simulink model "corr_test"  (Simulink 7.3)
settings: Solver=ode45  StartTime=0.0  StopTime=10000  RelTol=1e-3
libraries: xbsIndex_r4 x689, dali_library x32, dspsigops x2, xps_library x2, simulink x1, casper_library x1
(part 3 of 7)

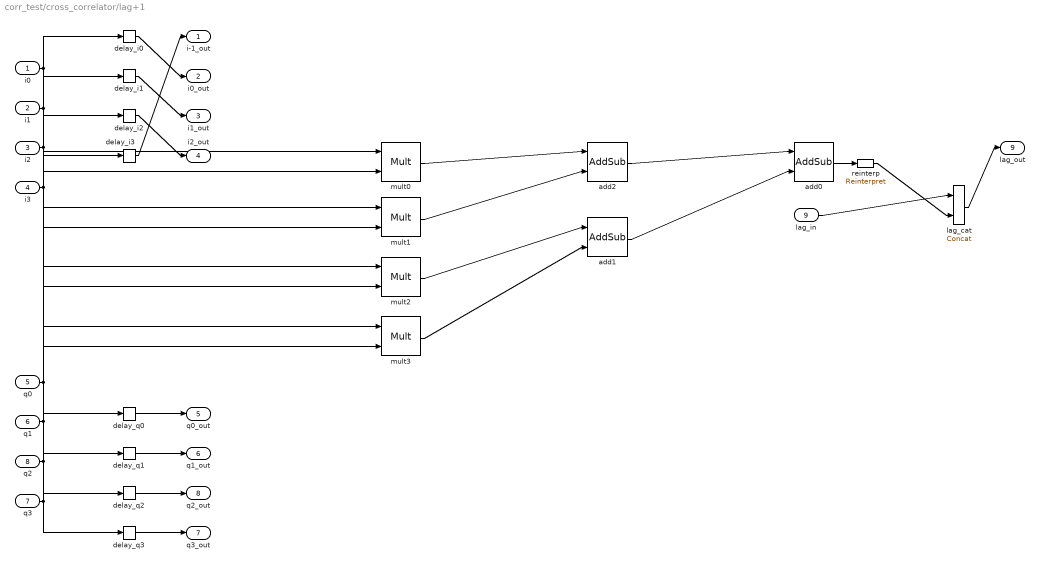
== system corr_test/cross_correlator/lag+1 ==
  i0 : Inport
  i1 : Inport  Port=2
  i2 : Inport  Port=3
  i3 : Inport  Port=4
  q0 : Inport  Port=5
  q1 : Inport  Port=6
  q3 : Inport  Port=7
  q2 : Inport  Port=8
  lag_in : Inport  Port=9
  add0 : xbsIndex_r4/AddSub  mode=Addition  use_carryin=off  use_carryout=off  en=off  latency=2  precision=Full  arith_type=Unsigned  n_bits=16  bin_pt=14  quantization=Truncate  overflow=Wrap  dbl_ovrd=off  use_behavioral_HDL=on  hw_selection=Fabric  pipelined=on  block_type=addsub
      settings: block_version=11.3
  add1 : xbsIndex_r4/AddSub  mode=Addition  use_carryin=off  use_carryout=off  en=off  latency=2  precision=Full  arith_type=Unsigned  n_bits=16  bin_pt=14  quantization=Truncate  overflow=Wrap  dbl_ovrd=off  use_behavioral_HDL=on  hw_selection=Fabric  pipelined=on  block_type=addsub
      settings: block_version=11.3
  add2 : xbsIndex_r4/AddSub  mode=Addition  use_carryin=off  use_carryout=off  en=off  latency=2  precision=Full  arith_type=Unsigned  n_bits=16  bin_pt=14  quantization=Truncate  overflow=Wrap  dbl_ovrd=off  use_behavioral_HDL=on  hw_selection=Fabric  pipelined=on  block_type=addsub
      settings: block_version=11.3
  delay_i0 : xbsIndex_r4/Delay  en=off  latency=0  dbl_ovrd=off  reg_retiming=off  block_type=delay
      settings: block_version=11.3
  delay_i1 : xbsIndex_r4/Delay  en=off  latency=0  dbl_ovrd=off  reg_retiming=off  block_type=delay
      settings: block_version=11.3
  delay_i2 : xbsIndex_r4/Delay  en=off  latency=0  dbl_ovrd=off  reg_retiming=off  block_type=delay
      settings: block_version=11.3
  delay_i3 : xbsIndex_r4/Delay  en=off  latency=1  dbl_ovrd=off  reg_retiming=off  block_type=delay
      settings: block_version=11.3
  delay_q{0..3} (4 alike) : xbsIndex_r4/Delay  en=off  latency=0  dbl_ovrd=off  reg_retiming=off  block_type=delay
      settings: block_version=11.3
  lag_cat : xbsIndex_r4/Concat  num_inputs=2  dbl_ovrd=off  block_type=concat
      settings: block_version=11.3
  mult{0..3} (4 alike) : xbsIndex_r4/Mult  precision=Full  arith_type="Signed  (2's comp)"  n_bits=16  bin_pt=14  quantization=Truncate  overflow=Wrap  en=off  latency=3  dbl_ovrd=off  use_behavioral_HDL=on  opt=Speed  use_embedded=off  optimum_pipeline=off  pipeline=on  use_rpm=on  placement_style=Triangular  block_type=mult
      settings: block_version=11.3
  reinterp : xbsIndex_r4/Reinterpret  force_arith_type=on  arith_type=Unsigned  force_bin_pt=on  bin_pt=0  block_type=reinterpret
      settings: infoedit="Changes signal type without altering the binary representation.   You can changed the signal between signed and unsigned, and relocate the binary point.<br><br>Hardware notes: In hardware this block costs nothing.<br><br>Example:  Suppose the input is 6 bits wide, signed, with 2 fractional bits, and the output is forced to unsigned with 0 fractional bits.  Then an input of -2.0 (1110.00 in binary 2's complement) becomes an output of 56 (111000 in binary)."  block_version=11.3
  i-1_out : Outport
  i0_out : Outport  Port=2
  i1_out : Outport  Port=3
  i2_out : Outport  Port=4
  q0_out : Outport  Port=5
  q1_out : Outport  Port=6
  q3_out : Outport  Port=7
  q2_out : Outport  Port=8
  lag_out : Outport  Port=9
  wires:
  i0/1 -> mult0/1, delay_i0/1
  q0/1 -> mult0/2, delay_q0/1
  i1/1 -> mult1/1, delay_i1/1
  q1/1 -> mult1/2, delay_q1/1
  i2/1 -> mult2/1, delay_i2/1
  q2/1 -> mult2/2, delay_q2/1
  i3/1 -> mult3/1, delay_i3/1
  q3/1 -> mult3/2, delay_q3/1
  mult0/1 -> add2/1
  mult1/1 -> add2/2
  mult2/1 -> add1/1
  mult3/1 -> add1/2
  add2/1 -> add0/1
  add1/1 -> add0/2
  delay_i0/1 -> i0_out/1
  delay_q0/1 -> q0_out/1
  delay_i1/1 -> i1_out/1
  delay_q1/1 -> q1_out/1
  delay_i2/1 -> i2_out/1
  delay_q2/1 -> q2_out/1
  delay_i3/1 -> i-1_out/1
  delay_q3/1 -> q3_out/1
  lag_in/1 -> lag_cat/1
  add0/1 -> reinterp/1
  reinterp/1 -> lag_cat/2
  lag_cat/1 -> lag_out/1

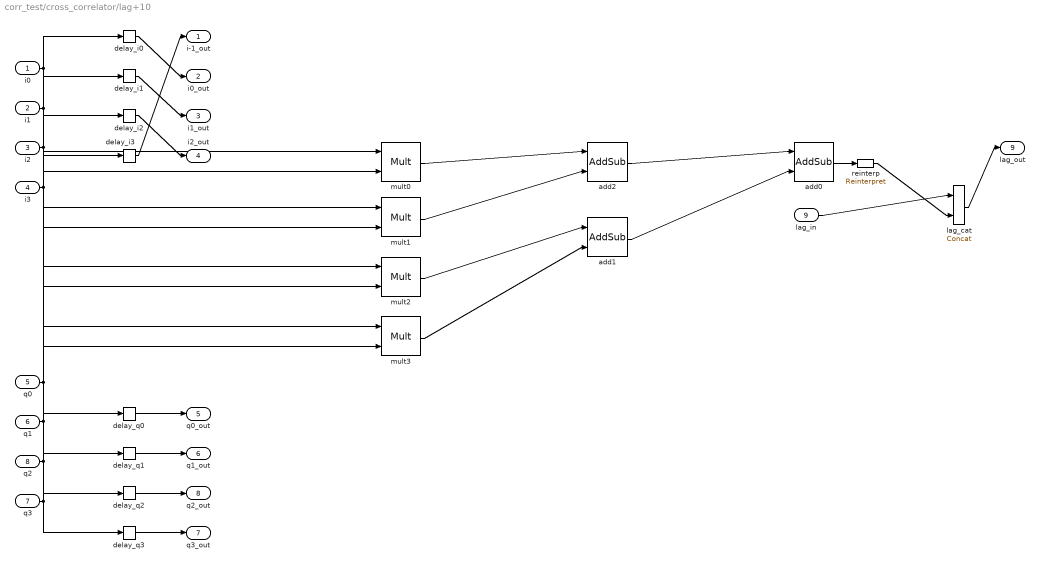
== system corr_test/cross_correlator/lag+10 ==
  i0 : Inport
  i1 : Inport  Port=2
  i2 : Inport  Port=3
  i3 : Inport  Port=4
  q0 : Inport  Port=5
  q1 : Inport  Port=6
  q3 : Inport  Port=7
  q2 : Inport  Port=8
  lag_in : Inport  Port=9
  add0 : xbsIndex_r4/AddSub  mode=Addition  use_carryin=off  use_carryout=off  en=off  latency=2  precision=Full  arith_type=Unsigned  n_bits=16  bin_pt=14  quantization=Truncate  overflow=Wrap  dbl_ovrd=off  use_behavioral_HDL=on  hw_selection=Fabric  pipelined=on  block_type=addsub
      settings: block_version=11.3
  add1 : xbsIndex_r4/AddSub  mode=Addition  use_carryin=off  use_carryout=off  en=off  latency=2  precision=Full  arith_type=Unsigned  n_bits=16  bin_pt=14  quantization=Truncate  overflow=Wrap  dbl_ovrd=off  use_behavioral_HDL=on  hw_selection=Fabric  pipelined=on  block_type=addsub
      settings: block_version=11.3
  add2 : xbsIndex_r4/AddSub  mode=Addition  use_carryin=off  use_carryout=off  en=off  latency=2  precision=Full  arith_type=Unsigned  n_bits=16  bin_pt=14  quantization=Truncate  overflow=Wrap  dbl_ovrd=off  use_behavioral_HDL=on  hw_selection=Fabric  pipelined=on  block_type=addsub
      settings: block_version=11.3
  delay_i0 : xbsIndex_r4/Delay  en=off  latency=0  dbl_ovrd=off  reg_retiming=off  block_type=delay
      settings: block_version=11.3
  delay_i1 : xbsIndex_r4/Delay  en=off  latency=0  dbl_ovrd=off  reg_retiming=off  block_type=delay
      settings: block_version=11.3
  delay_i2 : xbsIndex_r4/Delay  en=off  latency=0  dbl_ovrd=off  reg_retiming=off  block_type=delay
      settings: block_version=11.3
  delay_i3 : xbsIndex_r4/Delay  en=off  latency=1  dbl_ovrd=off  reg_retiming=off  block_type=delay
      settings: block_version=11.3
  delay_q{0..3} (4 alike) : xbsIndex_r4/Delay  en=off  latency=0  dbl_ovrd=off  reg_retiming=off  block_type=delay
      settings: block_version=11.3
  lag_cat : xbsIndex_r4/Concat  num_inputs=2  dbl_ovrd=off  block_type=concat
      settings: block_version=11.3
  mult{0..3} (4 alike) : xbsIndex_r4/Mult  precision=Full  arith_type="Signed  (2's comp)"  n_bits=16  bin_pt=14  quantization=Truncate  overflow=Wrap  en=off  latency=3  dbl_ovrd=off  use_behavioral_HDL=on  opt=Speed  use_embedded=off  optimum_pipeline=off  pipeline=on  use_rpm=on  placement_style=Triangular  block_type=mult
      settings: block_version=11.3
  reinterp : xbsIndex_r4/Reinterpret  force_arith_type=on  arith_type=Unsigned  force_bin_pt=on  bin_pt=0  block_type=reinterpret
      settings: infoedit="Changes signal type without altering the binary representation.   You can changed the signal between signed and unsigned, and relocate the binary point.<br><br>Hardware notes: In hardware this block costs nothing.<br><br>Example:  Suppose the input is 6 bits wide, signed, with 2 fractional bits, and the output is forced to unsigned with 0 fractional bits.  Then an input of -2.0 (1110.00 in binary 2's complement) becomes an output of 56 (111000 in binary)."  block_version=11.3
  i-1_out : Outport
  i0_out : Outport  Port=2
  i1_out : Outport  Port=3
  i2_out : Outport  Port=4
  q0_out : Outport  Port=5
  q1_out : Outport  Port=6
  q3_out : Outport  Port=7
  q2_out : Outport  Port=8
  lag_out : Outport  Port=9
  wires:
  i0/1 -> mult0/1, delay_i0/1
  q0/1 -> mult0/2, delay_q0/1
  i1/1 -> mult1/1, delay_i1/1
  q1/1 -> mult1/2, delay_q1/1
  i2/1 -> mult2/1, delay_i2/1
  q2/1 -> mult2/2, delay_q2/1
  i3/1 -> mult3/1, delay_i3/1
  q3/1 -> mult3/2, delay_q3/1
  mult0/1 -> add2/1
  mult1/1 -> add2/2
  mult2/1 -> add1/1
  mult3/1 -> add1/2
  add2/1 -> add0/1
  add1/1 -> add0/2
  delay_i0/1 -> i0_out/1
  delay_q0/1 -> q0_out/1
  delay_i1/1 -> i1_out/1
  delay_q1/1 -> q1_out/1
  delay_i2/1 -> i2_out/1
  delay_q2/1 -> q2_out/1
  delay_i3/1 -> i-1_out/1
  delay_q3/1 -> q3_out/1
  lag_in/1 -> lag_cat/1
  add0/1 -> reinterp/1
  reinterp/1 -> lag_cat/2
  lag_cat/1 -> lag_out/1

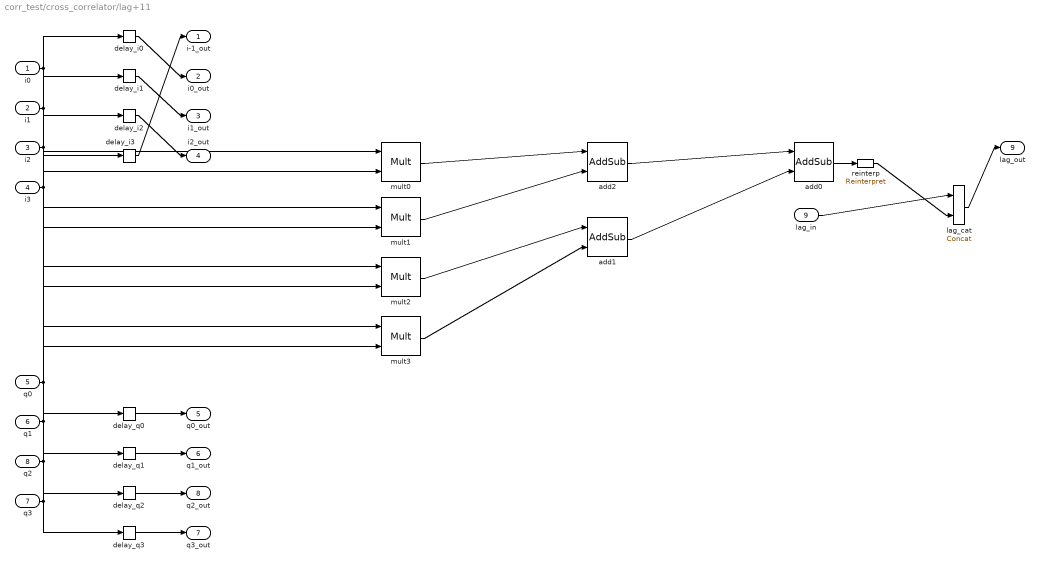
== system corr_test/cross_correlator/lag+11 ==
  i0 : Inport
  i1 : Inport  Port=2
  i2 : Inport  Port=3
  i3 : Inport  Port=4
  q0 : Inport  Port=5
  q1 : Inport  Port=6
  q3 : Inport  Port=7
  q2 : Inport  Port=8
  lag_in : Inport  Port=9
  add0 : xbsIndex_r4/AddSub  mode=Addition  use_carryin=off  use_carryout=off  en=off  latency=2  precision=Full  arith_type=Unsigned  n_bits=16  bin_pt=14  quantization=Truncate  overflow=Wrap  dbl_ovrd=off  use_behavioral_HDL=on  hw_selection=Fabric  pipelined=on  block_type=addsub
      settings: block_version=11.3
  add1 : xbsIndex_r4/AddSub  mode=Addition  use_carryin=off  use_carryout=off  en=off  latency=2  precision=Full  arith_type=Unsigned  n_bits=16  bin_pt=14  quantization=Truncate  overflow=Wrap  dbl_ovrd=off  use_behavioral_HDL=on  hw_selection=Fabric  pipelined=on  block_type=addsub
      settings: block_version=11.3
  add2 : xbsIndex_r4/AddSub  mode=Addition  use_carryin=off  use_carryout=off  en=off  latency=2  precision=Full  arith_type=Unsigned  n_bits=16  bin_pt=14  quantization=Truncate  overflow=Wrap  dbl_ovrd=off  use_behavioral_HDL=on  hw_selection=Fabric  pipelined=on  block_type=addsub
      settings: block_version=11.3
  delay_i0 : xbsIndex_r4/Delay  en=off  latency=0  dbl_ovrd=off  reg_retiming=off  block_type=delay
      settings: block_version=11.3
  delay_i1 : xbsIndex_r4/Delay  en=off  latency=0  dbl_ovrd=off  reg_retiming=off  block_type=delay
      settings: block_version=11.3
  delay_i2 : xbsIndex_r4/Delay  en=off  latency=0  dbl_ovrd=off  reg_retiming=off  block_type=delay
      settings: block_version=11.3
  delay_i3 : xbsIndex_r4/Delay  en=off  latency=1  dbl_ovrd=off  reg_retiming=off  block_type=delay
      settings: block_version=11.3
  delay_q{0..3} (4 alike) : xbsIndex_r4/Delay  en=off  latency=0  dbl_ovrd=off  reg_retiming=off  block_type=delay
      settings: block_version=11.3
  lag_cat : xbsIndex_r4/Concat  num_inputs=2  dbl_ovrd=off  block_type=concat
      settings: block_version=11.3
  mult{0..3} (4 alike) : xbsIndex_r4/Mult  precision=Full  arith_type="Signed  (2's comp)"  n_bits=16  bin_pt=14  quantization=Truncate  overflow=Wrap  en=off  latency=3  dbl_ovrd=off  use_behavioral_HDL=on  opt=Speed  use_embedded=off  optimum_pipeline=off  pipeline=on  use_rpm=on  placement_style=Triangular  block_type=mult
      settings: block_version=11.3
  reinterp : xbsIndex_r4/Reinterpret  force_arith_type=on  arith_type=Unsigned  force_bin_pt=on  bin_pt=0  block_type=reinterpret
      settings: infoedit="Changes signal type without altering the binary representation.   You can changed the signal between signed and unsigned, and relocate the binary point.<br><br>Hardware notes: In hardware this block costs nothing.<br><br>Example:  Suppose the input is 6 bits wide, signed, with 2 fractional bits, and the output is forced to unsigned with 0 fractional bits.  Then an input of -2.0 (1110.00 in binary 2's complement) becomes an output of 56 (111000 in binary)."  block_version=11.3
  i-1_out : Outport
  i0_out : Outport  Port=2
  i1_out : Outport  Port=3
  i2_out : Outport  Port=4
  q0_out : Outport  Port=5
  q1_out : Outport  Port=6
  q3_out : Outport  Port=7
  q2_out : Outport  Port=8
  lag_out : Outport  Port=9
  wires:
  i0/1 -> mult0/1, delay_i0/1
  q0/1 -> mult0/2, delay_q0/1
  i1/1 -> mult1/1, delay_i1/1
  q1/1 -> mult1/2, delay_q1/1
  i2/1 -> mult2/1, delay_i2/1
  q2/1 -> mult2/2, delay_q2/1
  i3/1 -> mult3/1, delay_i3/1
  q3/1 -> mult3/2, delay_q3/1
  mult0/1 -> add2/1
  mult1/1 -> add2/2
  mult2/1 -> add1/1
  mult3/1 -> add1/2
  add2/1 -> add0/1
  add1/1 -> add0/2
  delay_i0/1 -> i0_out/1
  delay_q0/1 -> q0_out/1
  delay_i1/1 -> i1_out/1
  delay_q1/1 -> q1_out/1
  delay_i2/1 -> i2_out/1
  delay_q2/1 -> q2_out/1
  delay_i3/1 -> i-1_out/1
  delay_q3/1 -> q3_out/1
  lag_in/1 -> lag_cat/1
  add0/1 -> reinterp/1
  reinterp/1 -> lag_cat/2
  lag_cat/1 -> lag_out/1

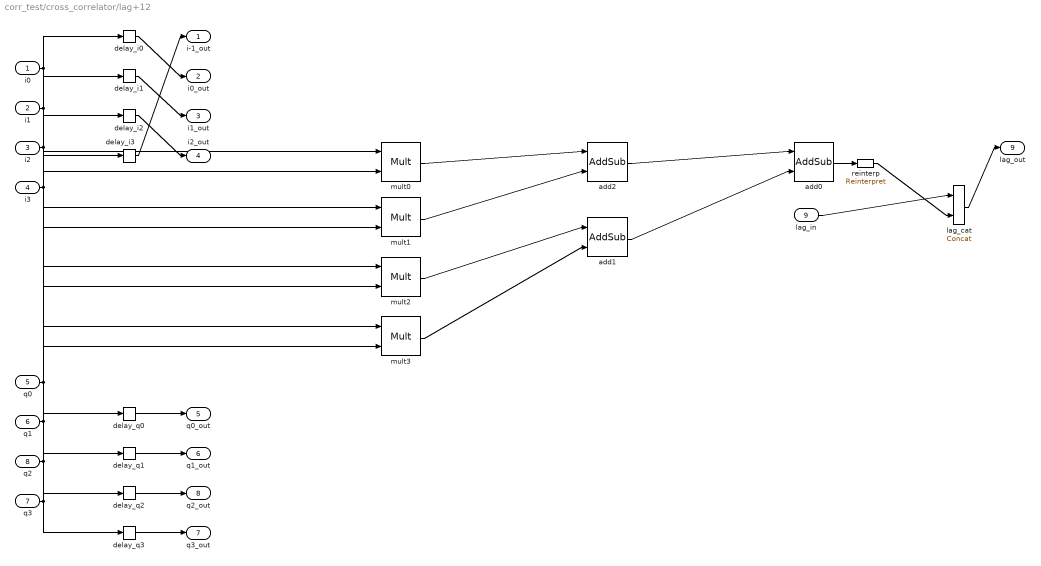
== system corr_test/cross_correlator/lag+12 ==
  i0 : Inport
  i1 : Inport  Port=2
  i2 : Inport  Port=3
  i3 : Inport  Port=4
  q0 : Inport  Port=5
  q1 : Inport  Port=6
  q3 : Inport  Port=7
  q2 : Inport  Port=8
  lag_in : Inport  Port=9
  add0 : xbsIndex_r4/AddSub  mode=Addition  use_carryin=off  use_carryout=off  en=off  latency=2  precision=Full  arith_type=Unsigned  n_bits=16  bin_pt=14  quantization=Truncate  overflow=Wrap  dbl_ovrd=off  use_behavioral_HDL=on  hw_selection=Fabric  pipelined=on  block_type=addsub
      settings: block_version=11.3
  add1 : xbsIndex_r4/AddSub  mode=Addition  use_carryin=off  use_carryout=off  en=off  latency=2  precision=Full  arith_type=Unsigned  n_bits=16  bin_pt=14  quantization=Truncate  overflow=Wrap  dbl_ovrd=off  use_behavioral_HDL=on  hw_selection=Fabric  pipelined=on  block_type=addsub
      settings: block_version=11.3
  add2 : xbsIndex_r4/AddSub  mode=Addition  use_carryin=off  use_carryout=off  en=off  latency=2  precision=Full  arith_type=Unsigned  n_bits=16  bin_pt=14  quantization=Truncate  overflow=Wrap  dbl_ovrd=off  use_behavioral_HDL=on  hw_selection=Fabric  pipelined=on  block_type=addsub
      settings: block_version=11.3
  delay_i0 : xbsIndex_r4/Delay  en=off  latency=0  dbl_ovrd=off  reg_retiming=off  block_type=delay
      settings: block_version=11.3
  delay_i1 : xbsIndex_r4/Delay  en=off  latency=0  dbl_ovrd=off  reg_retiming=off  block_type=delay
      settings: block_version=11.3
  delay_i2 : xbsIndex_r4/Delay  en=off  latency=0  dbl_ovrd=off  reg_retiming=off  block_type=delay
      settings: block_version=11.3
  delay_i3 : xbsIndex_r4/Delay  en=off  latency=1  dbl_ovrd=off  reg_retiming=off  block_type=delay
      settings: block_version=11.3
  delay_q{0..3} (4 alike) : xbsIndex_r4/Delay  en=off  latency=0  dbl_ovrd=off  reg_retiming=off  block_type=delay
      settings: block_version=11.3
  lag_cat : xbsIndex_r4/Concat  num_inputs=2  dbl_ovrd=off  block_type=concat
      settings: block_version=11.3
  mult{0..3} (4 alike) : xbsIndex_r4/Mult  precision=Full  arith_type="Signed  (2's comp)"  n_bits=16  bin_pt=14  quantization=Truncate  overflow=Wrap  en=off  latency=3  dbl_ovrd=off  use_behavioral_HDL=on  opt=Speed  use_embedded=off  optimum_pipeline=off  pipeline=on  use_rpm=on  placement_style=Triangular  block_type=mult
      settings: block_version=11.3
  reinterp : xbsIndex_r4/Reinterpret  force_arith_type=on  arith_type=Unsigned  force_bin_pt=on  bin_pt=0  block_type=reinterpret
      settings: infoedit="Changes signal type without altering the binary representation.   You can changed the signal between signed and unsigned, and relocate the binary point.<br><br>Hardware notes: In hardware this block costs nothing.<br><br>Example:  Suppose the input is 6 bits wide, signed, with 2 fractional bits, and the output is forced to unsigned with 0 fractional bits.  Then an input of -2.0 (1110.00 in binary 2's complement) becomes an output of 56 (111000 in binary)."  block_version=11.3
  i-1_out : Outport
  i0_out : Outport  Port=2
  i1_out : Outport  Port=3
  i2_out : Outport  Port=4
  q0_out : Outport  Port=5
  q1_out : Outport  Port=6
  q3_out : Outport  Port=7
  q2_out : Outport  Port=8
  lag_out : Outport  Port=9
  wires:
  i0/1 -> mult0/1, delay_i0/1
  q0/1 -> mult0/2, delay_q0/1
  i1/1 -> mult1/1, delay_i1/1
  q1/1 -> mult1/2, delay_q1/1
  i2/1 -> mult2/1, delay_i2/1
  q2/1 -> mult2/2, delay_q2/1
  i3/1 -> mult3/1, delay_i3/1
  q3/1 -> mult3/2, delay_q3/1
  mult0/1 -> add2/1
  mult1/1 -> add2/2
  mult2/1 -> add1/1
  mult3/1 -> add1/2
  add2/1 -> add0/1
  add1/1 -> add0/2
  delay_i0/1 -> i0_out/1
  delay_q0/1 -> q0_out/1
  delay_i1/1 -> i1_out/1
  delay_q1/1 -> q1_out/1
  delay_i2/1 -> i2_out/1
  delay_q2/1 -> q2_out/1
  delay_i3/1 -> i-1_out/1
  delay_q3/1 -> q3_out/1
  lag_in/1 -> lag_cat/1
  add0/1 -> reinterp/1
  reinterp/1 -> lag_cat/2
  lag_cat/1 -> lag_out/1

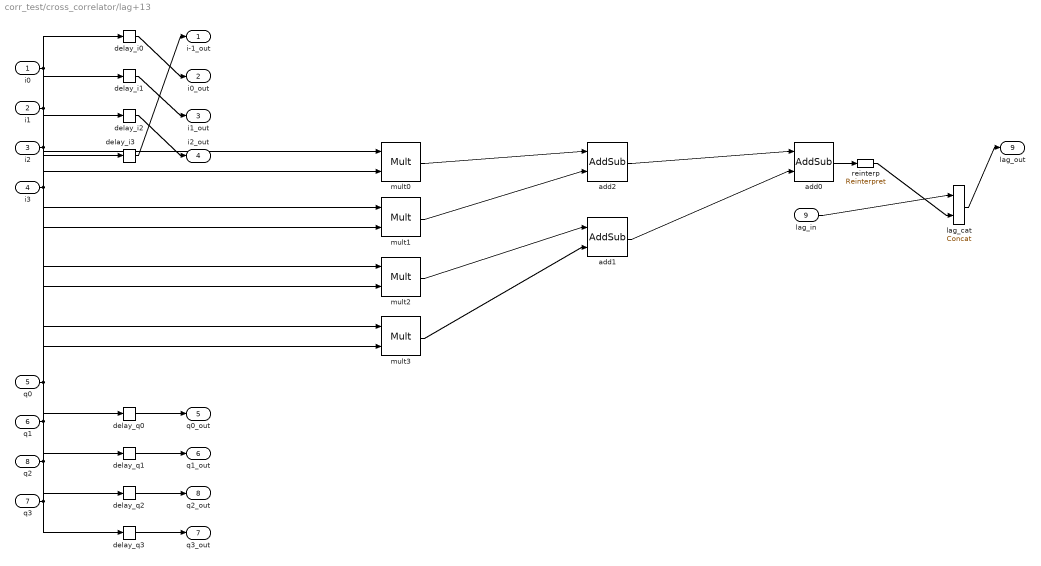
== system corr_test/cross_correlator/lag+13 ==
  i0 : Inport
  i1 : Inport  Port=2
  i2 : Inport  Port=3
  i3 : Inport  Port=4
  q0 : Inport  Port=5
  q1 : Inport  Port=6
  q3 : Inport  Port=7
  q2 : Inport  Port=8
  lag_in : Inport  Port=9
  add0 : xbsIndex_r4/AddSub  mode=Addition  use_carryin=off  use_carryout=off  en=off  latency=2  precision=Full  arith_type=Unsigned  n_bits=16  bin_pt=14  quantization=Truncate  overflow=Wrap  dbl_ovrd=off  use_behavioral_HDL=on  hw_selection=Fabric  pipelined=on  block_type=addsub
      settings: block_version=11.3
  add1 : xbsIndex_r4/AddSub  mode=Addition  use_carryin=off  use_carryout=off  en=off  latency=2  precision=Full  arith_type=Unsigned  n_bits=16  bin_pt=14  quantization=Truncate  overflow=Wrap  dbl_ovrd=off  use_behavioral_HDL=on  hw_selection=Fabric  pipelined=on  block_type=addsub
      settings: block_version=11.3
  add2 : xbsIndex_r4/AddSub  mode=Addition  use_carryin=off  use_carryout=off  en=off  latency=2  precision=Full  arith_type=Unsigned  n_bits=16  bin_pt=14  quantization=Truncate  overflow=Wrap  dbl_ovrd=off  use_behavioral_HDL=on  hw_selection=Fabric  pipelined=on  block_type=addsub
      settings: block_version=11.3
  delay_i0 : xbsIndex_r4/Delay  en=off  latency=0  dbl_ovrd=off  reg_retiming=off  block_type=delay
      settings: block_version=11.3
  delay_i1 : xbsIndex_r4/Delay  en=off  latency=0  dbl_ovrd=off  reg_retiming=off  block_type=delay
      settings: block_version=11.3
  delay_i2 : xbsIndex_r4/Delay  en=off  latency=0  dbl_ovrd=off  reg_retiming=off  block_type=delay
      settings: block_version=11.3
  delay_i3 : xbsIndex_r4/Delay  en=off  latency=1  dbl_ovrd=off  reg_retiming=off  block_type=delay
      settings: block_version=11.3
  delay_q{0..3} (4 alike) : xbsIndex_r4/Delay  en=off  latency=0  dbl_ovrd=off  reg_retiming=off  block_type=delay
      settings: block_version=11.3
  lag_cat : xbsIndex_r4/Concat  num_inputs=2  dbl_ovrd=off  block_type=concat
      settings: block_version=11.3
  mult{0..3} (4 alike) : xbsIndex_r4/Mult  precision=Full  arith_type="Signed  (2's comp)"  n_bits=16  bin_pt=14  quantization=Truncate  overflow=Wrap  en=off  latency=3  dbl_ovrd=off  use_behavioral_HDL=on  opt=Speed  use_embedded=off  optimum_pipeline=off  pipeline=on  use_rpm=on  placement_style=Triangular  block_type=mult
      settings: block_version=11.3
  reinterp : xbsIndex_r4/Reinterpret  force_arith_type=on  arith_type=Unsigned  force_bin_pt=on  bin_pt=0  block_type=reinterpret
      settings: infoedit="Changes signal type without altering the binary representation.   You can changed the signal between signed and unsigned, and relocate the binary point.<br><br>Hardware notes: In hardware this block costs nothing.<br><br>Example:  Suppose the input is 6 bits wide, signed, with 2 fractional bits, and the output is forced to unsigned with 0 fractional bits.  Then an input of -2.0 (1110.00 in binary 2's complement) becomes an output of 56 (111000 in binary)."  block_version=11.3
  i-1_out : Outport
  i0_out : Outport  Port=2
  i1_out : Outport  Port=3
  i2_out : Outport  Port=4
  q0_out : Outport  Port=5
  q1_out : Outport  Port=6
  q3_out : Outport  Port=7
  q2_out : Outport  Port=8
  lag_out : Outport  Port=9
  wires:
  i0/1 -> mult0/1, delay_i0/1
  q0/1 -> mult0/2, delay_q0/1
  i1/1 -> mult1/1, delay_i1/1
  q1/1 -> mult1/2, delay_q1/1
  i2/1 -> mult2/1, delay_i2/1
  q2/1 -> mult2/2, delay_q2/1
  i3/1 -> mult3/1, delay_i3/1
  q3/1 -> mult3/2, delay_q3/1
  mult0/1 -> add2/1
  mult1/1 -> add2/2
  mult2/1 -> add1/1
  mult3/1 -> add1/2
  add2/1 -> add0/1
  add1/1 -> add0/2
  delay_i0/1 -> i0_out/1
  delay_q0/1 -> q0_out/1
  delay_i1/1 -> i1_out/1
  delay_q1/1 -> q1_out/1
  delay_i2/1 -> i2_out/1
  delay_q2/1 -> q2_out/1
  delay_i3/1 -> i-1_out/1
  delay_q3/1 -> q3_out/1
  lag_in/1 -> lag_cat/1
  add0/1 -> reinterp/1
  reinterp/1 -> lag_cat/2
  lag_cat/1 -> lag_out/1

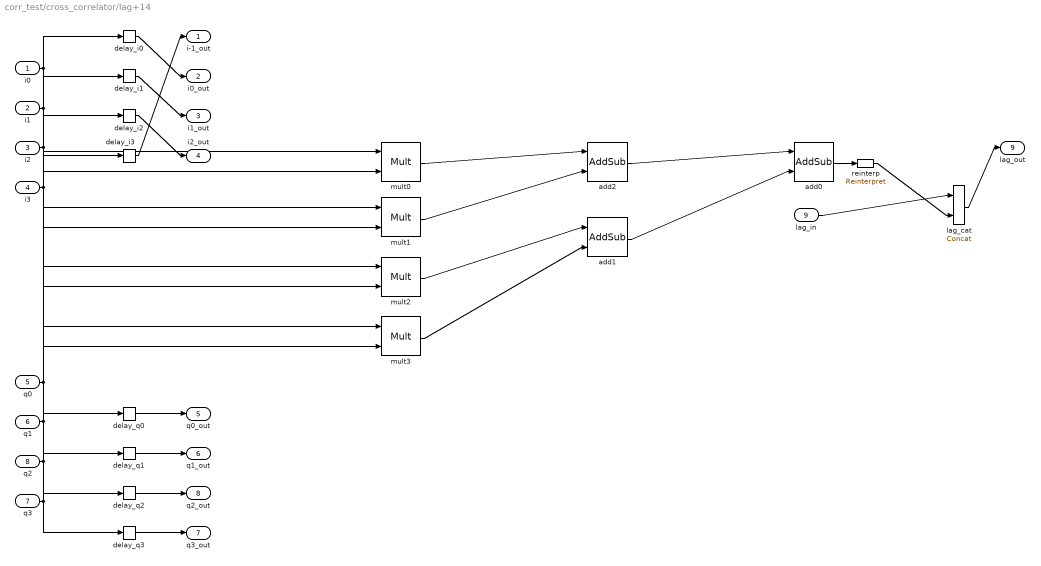
== system corr_test/cross_correlator/lag+14 ==
  i0 : Inport
  i1 : Inport  Port=2
  i2 : Inport  Port=3
  i3 : Inport  Port=4
  q0 : Inport  Port=5
  q1 : Inport  Port=6
  q3 : Inport  Port=7
  q2 : Inport  Port=8
  lag_in : Inport  Port=9
  add0 : xbsIndex_r4/AddSub  mode=Addition  use_carryin=off  use_carryout=off  en=off  latency=2  precision=Full  arith_type=Unsigned  n_bits=16  bin_pt=14  quantization=Truncate  overflow=Wrap  dbl_ovrd=off  use_behavioral_HDL=on  hw_selection=Fabric  pipelined=on  block_type=addsub
      settings: block_version=11.3
  add1 : xbsIndex_r4/AddSub  mode=Addition  use_carryin=off  use_carryout=off  en=off  latency=2  precision=Full  arith_type=Unsigned  n_bits=16  bin_pt=14  quantization=Truncate  overflow=Wrap  dbl_ovrd=off  use_behavioral_HDL=on  hw_selection=Fabric  pipelined=on  block_type=addsub
      settings: block_version=11.3
  add2 : xbsIndex_r4/AddSub  mode=Addition  use_carryin=off  use_carryout=off  en=off  latency=2  precision=Full  arith_type=Unsigned  n_bits=16  bin_pt=14  quantization=Truncate  overflow=Wrap  dbl_ovrd=off  use_behavioral_HDL=on  hw_selection=Fabric  pipelined=on  block_type=addsub
      settings: block_version=11.3
  delay_i0 : xbsIndex_r4/Delay  en=off  latency=0  dbl_ovrd=off  reg_retiming=off  block_type=delay
      settings: block_version=11.3
  delay_i1 : xbsIndex_r4/Delay  en=off  latency=0  dbl_ovrd=off  reg_retiming=off  block_type=delay
      settings: block_version=11.3
  delay_i2 : xbsIndex_r4/Delay  en=off  latency=0  dbl_ovrd=off  reg_retiming=off  block_type=delay
      settings: block_version=11.3
  delay_i3 : xbsIndex_r4/Delay  en=off  latency=1  dbl_ovrd=off  reg_retiming=off  block_type=delay
      settings: block_version=11.3
  delay_q{0..3} (4 alike) : xbsIndex_r4/Delay  en=off  latency=0  dbl_ovrd=off  reg_retiming=off  block_type=delay
      settings: block_version=11.3
  lag_cat : xbsIndex_r4/Concat  num_inputs=2  dbl_ovrd=off  block_type=concat
      settings: block_version=11.3
  mult{0..3} (4 alike) : xbsIndex_r4/Mult  precision=Full  arith_type="Signed  (2's comp)"  n_bits=16  bin_pt=14  quantization=Truncate  overflow=Wrap  en=off  latency=3  dbl_ovrd=off  use_behavioral_HDL=on  opt=Speed  use_embedded=off  optimum_pipeline=off  pipeline=on  use_rpm=on  placement_style=Triangular  block_type=mult
      settings: block_version=11.3
  reinterp : xbsIndex_r4/Reinterpret  force_arith_type=on  arith_type=Unsigned  force_bin_pt=on  bin_pt=0  block_type=reinterpret
      settings: infoedit="Changes signal type without altering the binary representation.   You can changed the signal between signed and unsigned, and relocate the binary point.<br><br>Hardware notes: In hardware this block costs nothing.<br><br>Example:  Suppose the input is 6 bits wide, signed, with 2 fractional bits, and the output is forced to unsigned with 0 fractional bits.  Then an input of -2.0 (1110.00 in binary 2's complement) becomes an output of 56 (111000 in binary)."  block_version=11.3
  i-1_out : Outport
  i0_out : Outport  Port=2
  i1_out : Outport  Port=3
  i2_out : Outport  Port=4
  q0_out : Outport  Port=5
  q1_out : Outport  Port=6
  q3_out : Outport  Port=7
  q2_out : Outport  Port=8
  lag_out : Outport  Port=9
  wires:
  i0/1 -> mult0/1, delay_i0/1
  q0/1 -> mult0/2, delay_q0/1
  i1/1 -> mult1/1, delay_i1/1
  q1/1 -> mult1/2, delay_q1/1
  i2/1 -> mult2/1, delay_i2/1
  q2/1 -> mult2/2, delay_q2/1
  i3/1 -> mult3/1, delay_i3/1
  q3/1 -> mult3/2, delay_q3/1
  mult0/1 -> add2/1
  mult1/1 -> add2/2
  mult2/1 -> add1/1
  mult3/1 -> add1/2
  add2/1 -> add0/1
  add1/1 -> add0/2
  delay_i0/1 -> i0_out/1
  delay_q0/1 -> q0_out/1
  delay_i1/1 -> i1_out/1
  delay_q1/1 -> q1_out/1
  delay_i2/1 -> i2_out/1
  delay_q2/1 -> q2_out/1
  delay_i3/1 -> i-1_out/1
  delay_q3/1 -> q3_out/1
  lag_in/1 -> lag_cat/1
  add0/1 -> reinterp/1
  reinterp/1 -> lag_cat/2
  lag_cat/1 -> lag_out/1

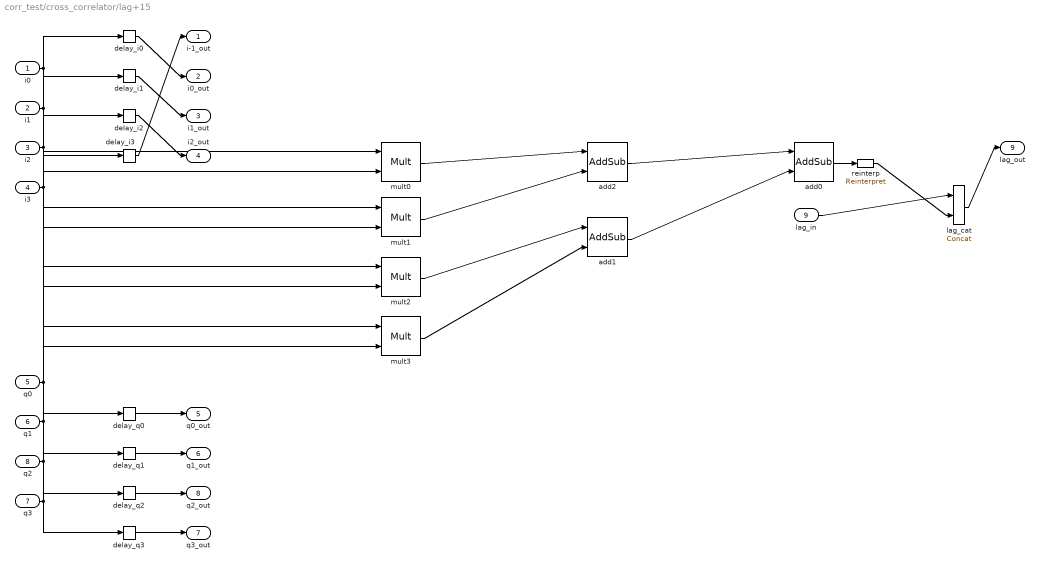
== system corr_test/cross_correlator/lag+15 ==
  i0 : Inport
  i1 : Inport  Port=2
  i2 : Inport  Port=3
  i3 : Inport  Port=4
  q0 : Inport  Port=5
  q1 : Inport  Port=6
  q3 : Inport  Port=7
  q2 : Inport  Port=8
  lag_in : Inport  Port=9
  add0 : xbsIndex_r4/AddSub  mode=Addition  use_carryin=off  use_carryout=off  en=off  latency=2  precision=Full  arith_type=Unsigned  n_bits=16  bin_pt=14  quantization=Truncate  overflow=Wrap  dbl_ovrd=off  use_behavioral_HDL=on  hw_selection=Fabric  pipelined=on  block_type=addsub
      settings: block_version=11.3
  add1 : xbsIndex_r4/AddSub  mode=Addition  use_carryin=off  use_carryout=off  en=off  latency=2  precision=Full  arith_type=Unsigned  n_bits=16  bin_pt=14  quantization=Truncate  overflow=Wrap  dbl_ovrd=off  use_behavioral_HDL=on  hw_selection=Fabric  pipelined=on  block_type=addsub
      settings: block_version=11.3
  add2 : xbsIndex_r4/AddSub  mode=Addition  use_carryin=off  use_carryout=off  en=off  latency=2  precision=Full  arith_type=Unsigned  n_bits=16  bin_pt=14  quantization=Truncate  overflow=Wrap  dbl_ovrd=off  use_behavioral_HDL=on  hw_selection=Fabric  pipelined=on  block_type=addsub
      settings: block_version=11.3
  delay_i0 : xbsIndex_r4/Delay  en=off  latency=0  dbl_ovrd=off  reg_retiming=off  block_type=delay
      settings: block_version=11.3
  delay_i1 : xbsIndex_r4/Delay  en=off  latency=0  dbl_ovrd=off  reg_retiming=off  block_type=delay
      settings: block_version=11.3
  delay_i2 : xbsIndex_r4/Delay  en=off  latency=0  dbl_ovrd=off  reg_retiming=off  block_type=delay
      settings: block_version=11.3
  delay_i3 : xbsIndex_r4/Delay  en=off  latency=1  dbl_ovrd=off  reg_retiming=off  block_type=delay
      settings: block_version=11.3
  delay_q{0..3} (4 alike) : xbsIndex_r4/Delay  en=off  latency=0  dbl_ovrd=off  reg_retiming=off  block_type=delay
      settings: block_version=11.3
  lag_cat : xbsIndex_r4/Concat  num_inputs=2  dbl_ovrd=off  block_type=concat
      settings: block_version=11.3
  mult{0..3} (4 alike) : xbsIndex_r4/Mult  precision=Full  arith_type="Signed  (2's comp)"  n_bits=16  bin_pt=14  quantization=Truncate  overflow=Wrap  en=off  latency=3  dbl_ovrd=off  use_behavioral_HDL=on  opt=Speed  use_embedded=off  optimum_pipeline=off  pipeline=on  use_rpm=on  placement_style=Triangular  block_type=mult
      settings: block_version=11.3
  reinterp : xbsIndex_r4/Reinterpret  force_arith_type=on  arith_type=Unsigned  force_bin_pt=on  bin_pt=0  block_type=reinterpret
      settings: infoedit="Changes signal type without altering the binary representation.   You can changed the signal between signed and unsigned, and relocate the binary point.<br><br>Hardware notes: In hardware this block costs nothing.<br><br>Example:  Suppose the input is 6 bits wide, signed, with 2 fractional bits, and the output is forced to unsigned with 0 fractional bits.  Then an input of -2.0 (1110.00 in binary 2's complement) becomes an output of 56 (111000 in binary)."  block_version=11.3
  i-1_out : Outport
  i0_out : Outport  Port=2
  i1_out : Outport  Port=3
  i2_out : Outport  Port=4
  q0_out : Outport  Port=5
  q1_out : Outport  Port=6
  q3_out : Outport  Port=7
  q2_out : Outport  Port=8
  lag_out : Outport  Port=9
  wires:
  i0/1 -> mult0/1, delay_i0/1
  q0/1 -> mult0/2, delay_q0/1
  i1/1 -> mult1/1, delay_i1/1
  q1/1 -> mult1/2, delay_q1/1
  i2/1 -> mult2/1, delay_i2/1
  q2/1 -> mult2/2, delay_q2/1
  i3/1 -> mult3/1, delay_i3/1
  q3/1 -> mult3/2, delay_q3/1
  mult0/1 -> add2/1
  mult1/1 -> add2/2
  mult2/1 -> add1/1
  mult3/1 -> add1/2
  add2/1 -> add0/1
  add1/1 -> add0/2
  delay_i0/1 -> i0_out/1
  delay_q0/1 -> q0_out/1
  delay_i1/1 -> i1_out/1
  delay_q1/1 -> q1_out/1
  delay_i2/1 -> i2_out/1
  delay_q2/1 -> q2_out/1
  delay_i3/1 -> i-1_out/1
  delay_q3/1 -> q3_out/1
  lag_in/1 -> lag_cat/1
  add0/1 -> reinterp/1
  reinterp/1 -> lag_cat/2
  lag_cat/1 -> lag_out/1

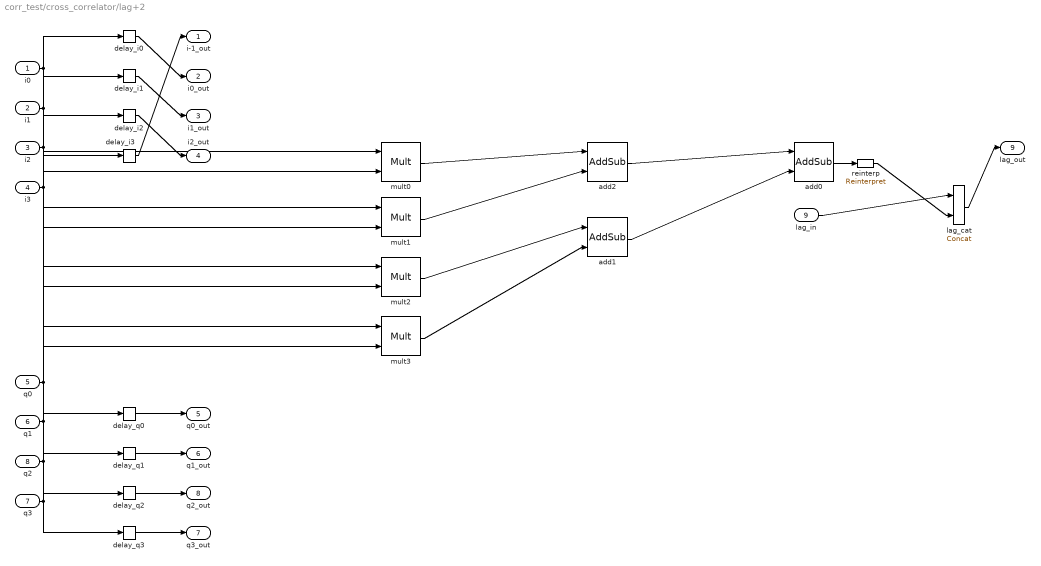
== system corr_test/cross_correlator/lag+2 ==
  i0 : Inport
  i1 : Inport  Port=2
  i2 : Inport  Port=3
  i3 : Inport  Port=4
  q0 : Inport  Port=5
  q1 : Inport  Port=6
  q3 : Inport  Port=7
  q2 : Inport  Port=8
  lag_in : Inport  Port=9
  add0 : xbsIndex_r4/AddSub  mode=Addition  use_carryin=off  use_carryout=off  en=off  latency=2  precision=Full  arith_type=Unsigned  n_bits=16  bin_pt=14  quantization=Truncate  overflow=Wrap  dbl_ovrd=off  use_behavioral_HDL=on  hw_selection=Fabric  pipelined=on  block_type=addsub
      settings: block_version=11.3
  add1 : xbsIndex_r4/AddSub  mode=Addition  use_carryin=off  use_carryout=off  en=off  latency=2  precision=Full  arith_type=Unsigned  n_bits=16  bin_pt=14  quantization=Truncate  overflow=Wrap  dbl_ovrd=off  use_behavioral_HDL=on  hw_selection=Fabric  pipelined=on  block_type=addsub
      settings: block_version=11.3
  add2 : xbsIndex_r4/AddSub  mode=Addition  use_carryin=off  use_carryout=off  en=off  latency=2  precision=Full  arith_type=Unsigned  n_bits=16  bin_pt=14  quantization=Truncate  overflow=Wrap  dbl_ovrd=off  use_behavioral_HDL=on  hw_selection=Fabric  pipelined=on  block_type=addsub
      settings: block_version=11.3
  delay_i0 : xbsIndex_r4/Delay  en=off  latency=0  dbl_ovrd=off  reg_retiming=off  block_type=delay
      settings: block_version=11.3
  delay_i1 : xbsIndex_r4/Delay  en=off  latency=0  dbl_ovrd=off  reg_retiming=off  block_type=delay
      settings: block_version=11.3
  delay_i2 : xbsIndex_r4/Delay  en=off  latency=0  dbl_ovrd=off  reg_retiming=off  block_type=delay
      settings: block_version=11.3
  delay_i3 : xbsIndex_r4/Delay  en=off  latency=1  dbl_ovrd=off  reg_retiming=off  block_type=delay
      settings: block_version=11.3
  delay_q{0..3} (4 alike) : xbsIndex_r4/Delay  en=off  latency=0  dbl_ovrd=off  reg_retiming=off  block_type=delay
      settings: block_version=11.3
  lag_cat : xbsIndex_r4/Concat  num_inputs=2  dbl_ovrd=off  block_type=concat
      settings: block_version=11.3
  mult{0..3} (4 alike) : xbsIndex_r4/Mult  precision=Full  arith_type="Signed  (2's comp)"  n_bits=16  bin_pt=14  quantization=Truncate  overflow=Wrap  en=off  latency=3  dbl_ovrd=off  use_behavioral_HDL=on  opt=Speed  use_embedded=off  optimum_pipeline=off  pipeline=on  use_rpm=on  placement_style=Triangular  block_type=mult
      settings: block_version=11.3
  reinterp : xbsIndex_r4/Reinterpret  force_arith_type=on  arith_type=Unsigned  force_bin_pt=on  bin_pt=0  block_type=reinterpret
      settings: infoedit="Changes signal type without altering the binary representation.   You can changed the signal between signed and unsigned, and relocate the binary point.<br><br>Hardware notes: In hardware this block costs nothing.<br><br>Example:  Suppose the input is 6 bits wide, signed, with 2 fractional bits, and the output is forced to unsigned with 0 fractional bits.  Then an input of -2.0 (1110.00 in binary 2's complement) becomes an output of 56 (111000 in binary)."  block_version=11.3
  i-1_out : Outport
  i0_out : Outport  Port=2
  i1_out : Outport  Port=3
  i2_out : Outport  Port=4
  q0_out : Outport  Port=5
  q1_out : Outport  Port=6
  q3_out : Outport  Port=7
  q2_out : Outport  Port=8
  lag_out : Outport  Port=9
  wires:
  i0/1 -> mult0/1, delay_i0/1
  q0/1 -> mult0/2, delay_q0/1
  i1/1 -> mult1/1, delay_i1/1
  q1/1 -> mult1/2, delay_q1/1
  i2/1 -> mult2/1, delay_i2/1
  q2/1 -> mult2/2, delay_q2/1
  i3/1 -> mult3/1, delay_i3/1
  q3/1 -> mult3/2, delay_q3/1
  mult0/1 -> add2/1
  mult1/1 -> add2/2
  mult2/1 -> add1/1
  mult3/1 -> add1/2
  add2/1 -> add0/1
  add1/1 -> add0/2
  delay_i0/1 -> i0_out/1
  delay_q0/1 -> q0_out/1
  delay_i1/1 -> i1_out/1
  delay_q1/1 -> q1_out/1
  delay_i2/1 -> i2_out/1
  delay_q2/1 -> q2_out/1
  delay_i3/1 -> i-1_out/1
  delay_q3/1 -> q3_out/1
  lag_in/1 -> lag_cat/1
  add0/1 -> reinterp/1
  reinterp/1 -> lag_cat/2
  lag_cat/1 -> lag_out/1

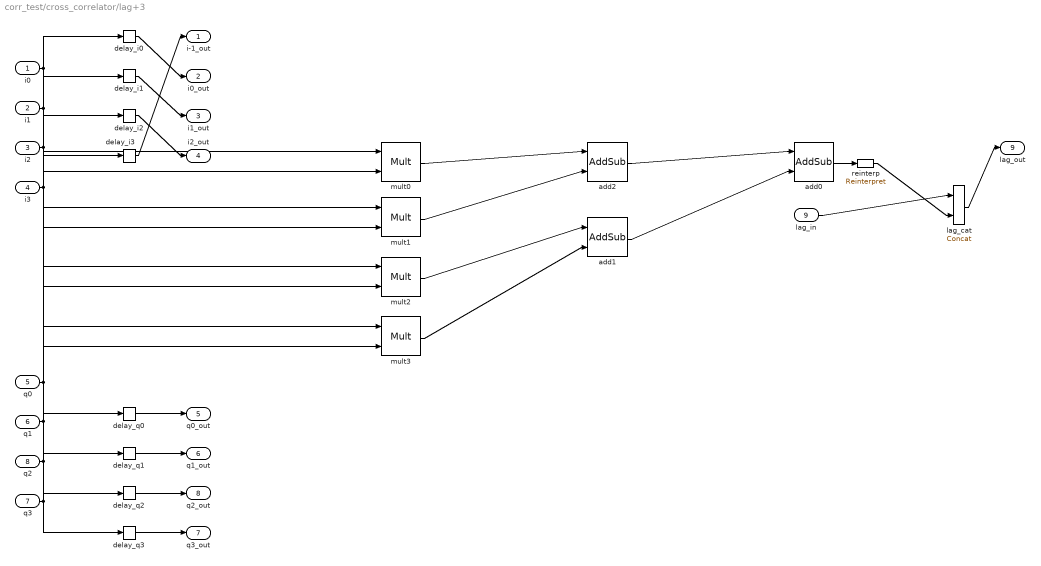
== system corr_test/cross_correlator/lag+3 ==
  i0 : Inport
  i1 : Inport  Port=2
  i2 : Inport  Port=3
  i3 : Inport  Port=4
  q0 : Inport  Port=5
  q1 : Inport  Port=6
  q3 : Inport  Port=7
  q2 : Inport  Port=8
  lag_in : Inport  Port=9
  add0 : xbsIndex_r4/AddSub  mode=Addition  use_carryin=off  use_carryout=off  en=off  latency=2  precision=Full  arith_type=Unsigned  n_bits=16  bin_pt=14  quantization=Truncate  overflow=Wrap  dbl_ovrd=off  use_behavioral_HDL=on  hw_selection=Fabric  pipelined=on  block_type=addsub
      settings: block_version=11.3
  add1 : xbsIndex_r4/AddSub  mode=Addition  use_carryin=off  use_carryout=off  en=off  latency=2  precision=Full  arith_type=Unsigned  n_bits=16  bin_pt=14  quantization=Truncate  overflow=Wrap  dbl_ovrd=off  use_behavioral_HDL=on  hw_selection=Fabric  pipelined=on  block_type=addsub
      settings: block_version=11.3
  add2 : xbsIndex_r4/AddSub  mode=Addition  use_carryin=off  use_carryout=off  en=off  latency=2  precision=Full  arith_type=Unsigned  n_bits=16  bin_pt=14  quantization=Truncate  overflow=Wrap  dbl_ovrd=off  use_behavioral_HDL=on  hw_selection=Fabric  pipelined=on  block_type=addsub
      settings: block_version=11.3
  delay_i0 : xbsIndex_r4/Delay  en=off  latency=0  dbl_ovrd=off  reg_retiming=off  block_type=delay
      settings: block_version=11.3
  delay_i1 : xbsIndex_r4/Delay  en=off  latency=0  dbl_ovrd=off  reg_retiming=off  block_type=delay
      settings: block_version=11.3
  delay_i2 : xbsIndex_r4/Delay  en=off  latency=0  dbl_ovrd=off  reg_retiming=off  block_type=delay
      settings: block_version=11.3
  delay_i3 : xbsIndex_r4/Delay  en=off  latency=1  dbl_ovrd=off  reg_retiming=off  block_type=delay
      settings: block_version=11.3
  delay_q{0..3} (4 alike) : xbsIndex_r4/Delay  en=off  latency=0  dbl_ovrd=off  reg_retiming=off  block_type=delay
      settings: block_version=11.3
  lag_cat : xbsIndex_r4/Concat  num_inputs=2  dbl_ovrd=off  block_type=concat
      settings: block_version=11.3
  mult{0..3} (4 alike) : xbsIndex_r4/Mult  precision=Full  arith_type="Signed  (2's comp)"  n_bits=16  bin_pt=14  quantization=Truncate  overflow=Wrap  en=off  latency=3  dbl_ovrd=off  use_behavioral_HDL=on  opt=Speed  use_embedded=off  optimum_pipeline=off  pipeline=on  use_rpm=on  placement_style=Triangular  block_type=mult
      settings: block_version=11.3
  reinterp : xbsIndex_r4/Reinterpret  force_arith_type=on  arith_type=Unsigned  force_bin_pt=on  bin_pt=0  block_type=reinterpret
      settings: infoedit="Changes signal type without altering the binary representation.   You can changed the signal between signed and unsigned, and relocate the binary point.<br><br>Hardware notes: In hardware this block costs nothing.<br><br>Example:  Suppose the input is 6 bits wide, signed, with 2 fractional bits, and the output is forced to unsigned with 0 fractional bits.  Then an input of -2.0 (1110.00 in binary 2's complement) becomes an output of 56 (111000 in binary)."  block_version=11.3
  i-1_out : Outport
  i0_out : Outport  Port=2
  i1_out : Outport  Port=3
  i2_out : Outport  Port=4
  q0_out : Outport  Port=5
  q1_out : Outport  Port=6
  q3_out : Outport  Port=7
  q2_out : Outport  Port=8
  lag_out : Outport  Port=9
  wires:
  i0/1 -> mult0/1, delay_i0/1
  q0/1 -> mult0/2, delay_q0/1
  i1/1 -> mult1/1, delay_i1/1
  q1/1 -> mult1/2, delay_q1/1
  i2/1 -> mult2/1, delay_i2/1
  q2/1 -> mult2/2, delay_q2/1
  i3/1 -> mult3/1, delay_i3/1
  q3/1 -> mult3/2, delay_q3/1
  mult0/1 -> add2/1
  mult1/1 -> add2/2
  mult2/1 -> add1/1
  mult3/1 -> add1/2
  add2/1 -> add0/1
  add1/1 -> add0/2
  delay_i0/1 -> i0_out/1
  delay_q0/1 -> q0_out/1
  delay_i1/1 -> i1_out/1
  delay_q1/1 -> q1_out/1
  delay_i2/1 -> i2_out/1
  delay_q2/1 -> q2_out/1
  delay_i3/1 -> i-1_out/1
  delay_q3/1 -> q3_out/1
  lag_in/1 -> lag_cat/1
  add0/1 -> reinterp/1
  reinterp/1 -> lag_cat/2
  lag_cat/1 -> lag_out/1

== system corr_test/cross_correlator/lag+4 ==
  i0 : Inport
  i1 : Inport  Port=2
  i2 : Inport  Port=3
  i3 : Inport  Port=4
  q0 : Inport  Port=5
  q1 : Inport  Port=6
  q3 : Inport  Port=7
  q2 : Inport  Port=8
  lag_in : Inport  Port=9
  add0 : xbsIndex_r4/AddSub  mode=Addition  use_carryin=off  use_carryout=off  en=off  latency=2  precision=Full  arith_type=Unsigned  n_bits=16  bin_pt=14  quantization=Truncate  overflow=Wrap  dbl_ovrd=off  use_behavioral_HDL=on  hw_selection=Fabric  pipelined=on  block_type=addsub
      settings: block_version=11.3
  add1 : xbsIndex_r4/AddSub  mode=Addition  use_carryin=off  use_carryout=off  en=off  latency=2  precision=Full  arith_type=Unsigned  n_bits=16  bin_pt=14  quantization=Truncate  overflow=Wrap  dbl_ovrd=off  use_behavioral_HDL=on  hw_selection=Fabric  pipelined=on  block_type=addsub
      settings: block_version=11.3
  add2 : xbsIndex_r4/AddSub  mode=Addition  use_carryin=off  use_carryout=off  en=off  latency=2  precision=Full  arith_type=Unsigned  n_bits=16  bin_pt=14  quantization=Truncate  overflow=Wrap  dbl_ovrd=off  use_behavioral_HDL=on  hw_selection=Fabric  pipelined=on  block_type=addsub
      settings: block_version=11.3
  delay_i0 : xbsIndex_r4/Delay  en=off  latency=0  dbl_ovrd=off  reg_retiming=off  block_type=delay
      settings: block_version=11.3
  delay_i1 : xbsIndex_r4/Delay  en=off  latency=0  dbl_ovrd=off  reg_retiming=off  block_type=delay
      settings: block_version=11.3
  delay_i2 : xbsIndex_r4/Delay  en=off  latency=0  dbl_ovrd=off  reg_retiming=off  block_type=delay
      settings: block_version=11.3
  delay_i3 : xbsIndex_r4/Delay  en=off  latency=1  dbl_ovrd=off  reg_retiming=off  block_type=delay
      settings: block_version=11.3
  delay_q{0..3} (4 alike) : xbsIndex_r4/Delay  en=off  latency=0  dbl_ovrd=off  reg_retiming=off  block_type=delay
      settings: block_version=11.3
  lag_cat : xbsIndex_r4/Concat  num_inputs=2  dbl_ovrd=off  block_type=concat
      settings: block_version=11.3
  mult{0..3} (4 alike) : xbsIndex_r4/Mult  precision=Full  arith_type="Signed  (2's comp)"  n_bits=16  bin_pt=14  quantization=Truncate  overflow=Wrap  en=off  latency=3  dbl_ovrd=off  use_behavioral_HDL=on  opt=Speed  use_embedded=off  optimum_pipeline=off  pipeline=on  use_rpm=on  placement_style=Triangular  block_type=mult
      settings: block_version=11.3
  reinterp : xbsIndex_r4/Reinterpret  force_arith_type=on  arith_type=Unsigned  force_bin_pt=on  bin_pt=0  block_type=reinterpret
      settings: infoedit="Changes signal type without altering the binary representation.   You can changed the signal between signed and unsigned, and relocate the binary point.<br><br>Hardware notes: In hardware this block costs nothing.<br><br>Example:  Suppose the input is 6 bits wide, signed, with 2 fractional bits, and the output is forced to unsigned with 0 fractional bits.  Then an input of -2.0 (1110.00 in binary 2's complement) becomes an output of 56 (111000 in binary)."  block_version=11.3
  i-1_out : Outport
  i0_out : Outport  Port=2
  i1_out : Outport  Port=3
  i2_out : Outport  Port=4
  q0_out : Outport  Port=5
  q1_out : Outport  Port=6
  q3_out : Outport  Port=7
  q2_out : Outport  Port=8
  lag_out : Outport  Port=9
  wires:
  i0/1 -> mult0/1, delay_i0/1
  q0/1 -> mult0/2, delay_q0/1
  i1/1 -> mult1/1, delay_i1/1
  q1/1 -> mult1/2, delay_q1/1
  i2/1 -> mult2/1, delay_i2/1
  q2/1 -> mult2/2, delay_q2/1
  i3/1 -> mult3/1, delay_i3/1
  q3/1 -> mult3/2, delay_q3/1
  mult0/1 -> add2/1
  mult1/1 -> add2/2
  mult2/1 -> add1/1
  mult3/1 -> add1/2
  add2/1 -> add0/1
  add1/1 -> add0/2
  delay_i0/1 -> i0_out/1
  delay_q0/1 -> q0_out/1
  delay_i1/1 -> i1_out/1
  delay_q1/1 -> q1_out/1
  delay_i2/1 -> i2_out/1
  delay_q2/1 -> q2_out/1
  delay_i3/1 -> i-1_out/1
  delay_q3/1 -> q3_out/1
  lag_in/1 -> lag_cat/1
  add0/1 -> reinterp/1
  reinterp/1 -> lag_cat/2
  lag_cat/1 -> lag_out/1

== system corr_test/cross_correlator/lag+5 ==
  i0 : Inport
  i1 : Inport  Port=2
  i2 : Inport  Port=3
  i3 : Inport  Port=4
  q0 : Inport  Port=5
  q1 : Inport  Port=6
  q3 : Inport  Port=7
  q2 : Inport  Port=8
  lag_in : Inport  Port=9
  add0 : xbsIndex_r4/AddSub  mode=Addition  use_carryin=off  use_carryout=off  en=off  latency=2  precision=Full  arith_type=Unsigned  n_bits=16  bin_pt=14  quantization=Truncate  overflow=Wrap  dbl_ovrd=off  use_behavioral_HDL=on  hw_selection=Fabric  pipelined=on  block_type=addsub
      settings: block_version=11.3
  add1 : xbsIndex_r4/AddSub  mode=Addition  use_carryin=off  use_carryout=off  en=off  latency=2  precision=Full  arith_type=Unsigned  n_bits=16  bin_pt=14  quantization=Truncate  overflow=Wrap  dbl_ovrd=off  use_behavioral_HDL=on  hw_selection=Fabric  pipelined=on  block_type=addsub
      settings: block_version=11.3
  add2 : xbsIndex_r4/AddSub  mode=Addition  use_carryin=off  use_carryout=off  en=off  latency=2  precision=Full  arith_type=Unsigned  n_bits=16  bin_pt=14  quantization=Truncate  overflow=Wrap  dbl_ovrd=off  use_behavioral_HDL=on  hw_selection=Fabric  pipelined=on  block_type=addsub
      settings: block_version=11.3
  delay_i0 : xbsIndex_r4/Delay  en=off  latency=0  dbl_ovrd=off  reg_retiming=off  block_type=delay
      settings: block_version=11.3
  delay_i1 : xbsIndex_r4/Delay  en=off  latency=0  dbl_ovrd=off  reg_retiming=off  block_type=delay
      settings: block_version=11.3
  delay_i2 : xbsIndex_r4/Delay  en=off  latency=0  dbl_ovrd=off  reg_retiming=off  block_type=delay
      settings: block_version=11.3
  delay_i3 : xbsIndex_r4/Delay  en=off  latency=1  dbl_ovrd=off  reg_retiming=off  block_type=delay
      settings: block_version=11.3
  delay_q{0..3} (4 alike) : xbsIndex_r4/Delay  en=off  latency=0  dbl_ovrd=off  reg_retiming=off  block_type=delay
      settings: block_version=11.3
  lag_cat : xbsIndex_r4/Concat  num_inputs=2  dbl_ovrd=off  block_type=concat
      settings: block_version=11.3
  mult{0..3} (4 alike) : xbsIndex_r4/Mult  precision=Full  arith_type="Signed  (2's comp)"  n_bits=16  bin_pt=14  quantization=Truncate  overflow=Wrap  en=off  latency=3  dbl_ovrd=off  use_behavioral_HDL=on  opt=Speed  use_embedded=off  optimum_pipeline=off  pipeline=on  use_rpm=on  placement_style=Triangular  block_type=mult
      settings: block_version=11.3
  reinterp : xbsIndex_r4/Reinterpret  force_arith_type=on  arith_type=Unsigned  force_bin_pt=on  bin_pt=0  block_type=reinterpret
      settings: infoedit="Changes signal type without altering the binary representation.   You can changed the signal between signed and unsigned, and relocate the binary point.<br><br>Hardware notes: In hardware this block costs nothing.<br><br>Example:  Suppose the input is 6 bits wide, signed, with 2 fractional bits, and the output is forced to unsigned with 0 fractional bits.  Then an input of -2.0 (1110.00 in binary 2's complement) becomes an output of 56 (111000 in binary)."  block_version=11.3
  i-1_out : Outport
  i0_out : Outport  Port=2
  i1_out : Outport  Port=3
  i2_out : Outport  Port=4
  q0_out : Outport  Port=5
  q1_out : Outport  Port=6
  q3_out : Outport  Port=7
  q2_out : Outport  Port=8
  lag_out : Outport  Port=9
  wires:
  i0/1 -> mult0/1, delay_i0/1
  q0/1 -> mult0/2, delay_q0/1
  i1/1 -> mult1/1, delay_i1/1
  q1/1 -> mult1/2, delay_q1/1
  i2/1 -> mult2/1, delay_i2/1
  q2/1 -> mult2/2, delay_q2/1
  i3/1 -> mult3/1, delay_i3/1
  q3/1 -> mult3/2, delay_q3/1
  mult0/1 -> add2/1
  mult1/1 -> add2/2
  mult2/1 -> add1/1
  mult3/1 -> add1/2
  add2/1 -> add0/1
  add1/1 -> add0/2
  delay_i0/1 -> i0_out/1
  delay_q0/1 -> q0_out/1
  delay_i1/1 -> i1_out/1
  delay_q1/1 -> q1_out/1
  delay_i2/1 -> i2_out/1
  delay_q2/1 -> q2_out/1
  delay_i3/1 -> i-1_out/1
  delay_q3/1 -> q3_out/1
  lag_in/1 -> lag_cat/1
  add0/1 -> reinterp/1
  reinterp/1 -> lag_cat/2
  lag_cat/1 -> lag_out/1

== system corr_test/cross_correlator/lag+6 ==
  i0 : Inport
  i1 : Inport  Port=2
  i2 : Inport  Port=3
  i3 : Inport  Port=4
  q0 : Inport  Port=5
  q1 : Inport  Port=6
  q3 : Inport  Port=7
  q2 : Inport  Port=8
  lag_in : Inport  Port=9
  add0 : xbsIndex_r4/AddSub  mode=Addition  use_carryin=off  use_carryout=off  en=off  latency=2  precision=Full  arith_type=Unsigned  n_bits=16  bin_pt=14  quantization=Truncate  overflow=Wrap  dbl_ovrd=off  use_behavioral_HDL=on  hw_selection=Fabric  pipelined=on  block_type=addsub
      settings: block_version=11.3
  add1 : xbsIndex_r4/AddSub  mode=Addition  use_carryin=off  use_carryout=off  en=off  latency=2  precision=Full  arith_type=Unsigned  n_bits=16  bin_pt=14  quantization=Truncate  overflow=Wrap  dbl_ovrd=off  use_behavioral_HDL=on  hw_selection=Fabric  pipelined=on  block_type=addsub
      settings: block_version=11.3
  add2 : xbsIndex_r4/AddSub  mode=Addition  use_carryin=off  use_carryout=off  en=off  latency=2  precision=Full  arith_type=Unsigned  n_bits=16  bin_pt=14  quantization=Truncate  overflow=Wrap  dbl_ovrd=off  use_behavioral_HDL=on  hw_selection=Fabric  pipelined=on  block_type=addsub
      settings: block_version=11.3
  delay_i0 : xbsIndex_r4/Delay  en=off  latency=0  dbl_ovrd=off  reg_retiming=off  block_type=delay
      settings: block_version=11.3
  delay_i1 : xbsIndex_r4/Delay  en=off  latency=0  dbl_ovrd=off  reg_retiming=off  block_type=delay
      settings: block_version=11.3
  delay_i2 : xbsIndex_r4/Delay  en=off  latency=0  dbl_ovrd=off  reg_retiming=off  block_type=delay
      settings: block_version=11.3
  delay_i3 : xbsIndex_r4/Delay  en=off  latency=1  dbl_ovrd=off  reg_retiming=off  block_type=delay
      settings: block_version=11.3
  delay_q{0..3} (4 alike) : xbsIndex_r4/Delay  en=off  latency=0  dbl_ovrd=off  reg_retiming=off  block_type=delay
      settings: block_version=11.3
  lag_cat : xbsIndex_r4/Concat  num_inputs=2  dbl_ovrd=off  block_type=concat
      settings: block_version=11.3
  mult{0..3} (4 alike) : xbsIndex_r4/Mult  precision=Full  arith_type="Signed  (2's comp)"  n_bits=16  bin_pt=14  quantization=Truncate  overflow=Wrap  en=off  latency=3  dbl_ovrd=off  use_behavioral_HDL=on  opt=Speed  use_embedded=off  optimum_pipeline=off  pipeline=on  use_rpm=on  placement_style=Triangular  block_type=mult
      settings: block_version=11.3
  reinterp : xbsIndex_r4/Reinterpret  force_arith_type=on  arith_type=Unsigned  force_bin_pt=on  bin_pt=0  block_type=reinterpret
      settings: infoedit="Changes signal type without altering the binary representation.   You can changed the signal between signed and unsigned, and relocate the binary point.<br><br>Hardware notes: In hardware this block costs nothing.<br><br>Example:  Suppose the input is 6 bits wide, signed, with 2 fractional bits, and the output is forced to unsigned with 0 fractional bits.  Then an input of -2.0 (1110.00 in binary 2's complement) becomes an output of 56 (111000 in binary)."  block_version=11.3
  i-1_out : Outport
  i0_out : Outport  Port=2
  i1_out : Outport  Port=3
  i2_out : Outport  Port=4
  q0_out : Outport  Port=5
  q1_out : Outport  Port=6
  q3_out : Outport  Port=7
  q2_out : Outport  Port=8
  lag_out : Outport  Port=9
  wires:
  i0/1 -> mult0/1, delay_i0/1
  q0/1 -> mult0/2, delay_q0/1
  i1/1 -> mult1/1, delay_i1/1
  q1/1 -> mult1/2, delay_q1/1
  i2/1 -> mult2/1, delay_i2/1
  q2/1 -> mult2/2, delay_q2/1
  i3/1 -> mult3/1, delay_i3/1
  q3/1 -> mult3/2, delay_q3/1
  mult0/1 -> add2/1
  mult1/1 -> add2/2
  mult2/1 -> add1/1
  mult3/1 -> add1/2
  add2/1 -> add0/1
  add1/1 -> add0/2
  delay_i0/1 -> i0_out/1
  delay_q0/1 -> q0_out/1
  delay_i1/1 -> i1_out/1
  delay_q1/1 -> q1_out/1
  delay_i2/1 -> i2_out/1
  delay_q2/1 -> q2_out/1
  delay_i3/1 -> i-1_out/1
  delay_q3/1 -> q3_out/1
  lag_in/1 -> lag_cat/1
  add0/1 -> reinterp/1
  reinterp/1 -> lag_cat/2
  lag_cat/1 -> lag_out/1
